simulink model "simsop"  (R2025a)
settings: Solver=VariableStepAuto  StartTime=0.0  StopTime=10.0  RelTol=1e-3
undefined symbols (not defined in the file or in its folder): dspblkCoreblockFVToolHelper, gcbh
libraries: simulink x3

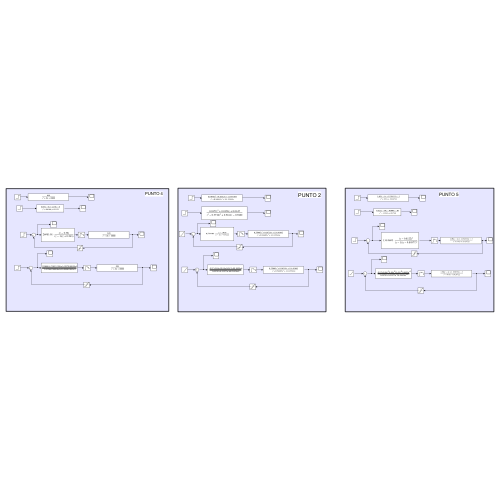
[thumbnail: Simulink's stored preview of the top-level diagram]
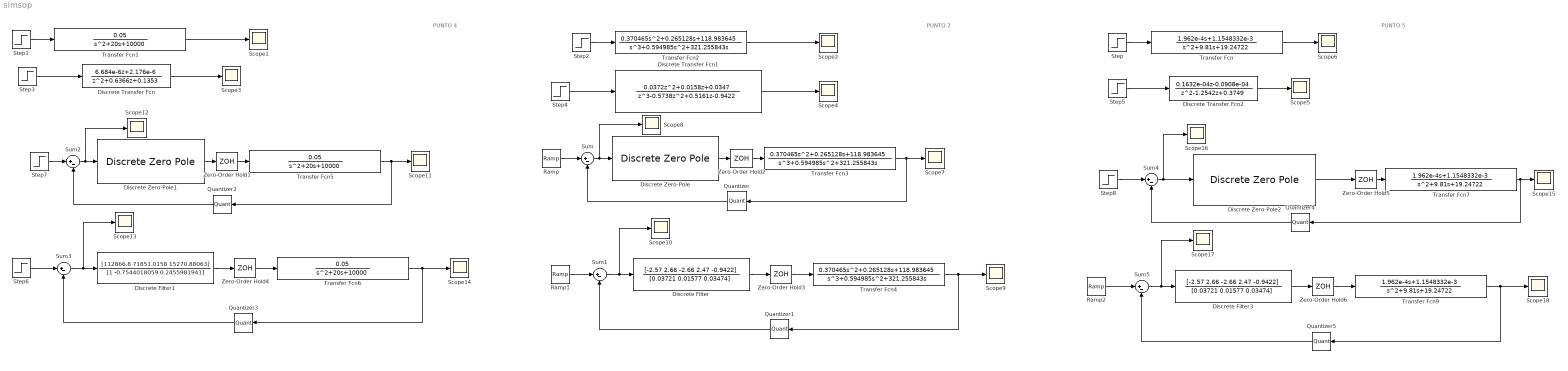
== system simsop ==
  note: PUNTO 5
  note: PUNTO 4
  note: PUNTO 2
  Discrete Transfer Fcn : DiscreteTransferFcn  LoadFcn=dspblkCoreblockFVToolHelper(gcbh,'load');  Numerator=[6.684e-6 2.176e-6]  Denominator=[1 0.6366 0.1353]
  Discrete Transfer Fcn1 : DiscreteTransferFcn  LoadFcn=dspblkCoreblockFVToolHelper(gcbh,'load');  Numerator="[0.0372    0.0158    0.0347]"  Denominator="[1   -0.5738    0.5161   -0.9422]"
  Discrete Transfer Fcn2 : DiscreteTransferFcn  LoadFcn=dspblkCoreblockFVToolHelper(gcbh,'load');  Numerator="[0.1632e-04   -0.0908e-04]"  Denominator="[1 -1.2542    0.3749]"
  Discrete Zero-Pole : DiscreteZeroPole  Zeros=[1.016]  Poles=[1 0.8222]  Gain=0.5798809  SampleTime=-1
  Discrete Zero-Pole1 : DiscreteZeroPole  Zeros=[2.52]  Poles=[1 -0.243]  Gain=26983.01  SampleTime=-1
  Discrete Zero-Pole2 : DiscreteZeroPole  Zeros=[0.8122 0.8122]  Poles=[1 0.80577 0.80577]  Gain=133.0695  SampleTime=-1
  Discrete Filter : DiscreteFilter  LoadFcn=dspblkCoreblockFVToolHelper(gcbh,'load');  Numerator=[-2.57 2.66 -2.66 2.47 -0.9422]  Denominator=[0.03721 0.01577 0.03474]
  Discrete Filter1 : DiscreteFilter  LoadFcn=dspblkCoreblockFVToolHelper(gcbh,'load');  Numerator=[112866.8 71851.0158 15270.88063]  Denominator=[1 -0.7544018059 0.2455981941]
  Discrete Filter3 : DiscreteFilter  LoadFcn=dspblkCoreblockFVToolHelper(gcbh,'load');  Numerator=[-2.57 2.66 -2.66 2.47 -0.9422]  Denominator=[0.03721 0.01577 0.03474]
  Quantizer{,1..5} (6 alike) : Quantizer  QuantizationInterval=3.3/1024
  Ramp : simulink/Sources/Ramp  slope=1  start=0  InitialOutput=0
  Ramp1 : simulink/Sources/Ramp  slope=1  start=0  InitialOutput=0
  Ramp2 : simulink/Sources/Ramp  slope=1  start=0  InitialOutput=0
  Scope{1..18} (18 alike) : Scope
  Step{,1..8} (9 alike) : Step  Time=0  SampleTime=0
  Sum{,1..5} (6 alike) : Sum  Inputs=|+-
  Transfer Fcn : TransferFcn  Numerator=[1.962e-4 1.1548332e-3]  Denominator=[1 9.81 19.24722]
  Transfer Fcn1 : TransferFcn  Numerator=[0.05]  Denominator=[1 20 10000]
  Transfer Fcn2 : TransferFcn  Numerator=[0.370465 0.265128 118.983645]  Denominator=[1 0.594985 321.255843 0]
  Transfer Fcn3 : TransferFcn  Numerator=[0.370465 0.265128 118.983645]  Denominator=[1 0.594985 321.255843 0]
  Transfer Fcn4 : TransferFcn  Numerator=[0.370465 0.265128 118.983645]  Denominator=[1 0.594985 321.255843 0]
  Transfer Fcn5 : TransferFcn  Numerator=[0.05]  Denominator=[1 20 10000]
  Transfer Fcn6 : TransferFcn  Numerator=[0.05]  Denominator=[1 20 10000]
  Transfer Fcn7 : TransferFcn  Numerator=[1.962e-4 1.1548332e-3]  Denominator=[1 9.81 19.24722]
  Transfer Fcn9 : TransferFcn  Numerator=[1.962e-4 1.1548332e-3]  Denominator=[1 9.81 19.24722]
  Zero-Order Hold{1..6} (6 alike) : ZeroOrderHold  SampleTime=0.1
  wires:
  Transfer Fcn/1 -> Scope6/1
  Step1/1 -> Transfer Fcn1/1
  Step2/1 -> Transfer Fcn2/1
  Discrete Transfer Fcn/1 -> Scope3/1
  Transfer Fcn1/1 -> Scope1/1
  Step3/1 -> Discrete Transfer Fcn/1
  Step4/1 -> Discrete Transfer Fcn1/1
  Transfer Fcn2/1 -> Scope2/1
  Discrete Transfer Fcn1/1 -> Scope4/1
  Discrete Transfer Fcn2/1 -> Scope5/1
  Discrete Zero-Pole/1 -> Zero-Order Hold2/1
  Quantizer/1 -> Sum/2
  Sum/1 -> Discrete Zero-Pole/1, Scope8/1
  Transfer Fcn3/1 -> Scope7/1, Quantizer/1
  Ramp/1 -> Sum/1
  Zero-Order Hold2/1 -> Transfer Fcn3/1
  Discrete Filter/1 -> Zero-Order Hold3/1
  Quantizer1/1 -> Sum1/2
  Zero-Order Hold3/1 -> Transfer Fcn4/1
  Sum1/1 -> Scope10/1, Discrete Filter/1
  Transfer Fcn4/1 -> Scope9/1, Quantizer1/1
  Ramp1/1 -> Sum1/1
  Zero-Order Hold1/1 -> Transfer Fcn5/1
  Step7/1 -> Sum2/1
  Transfer Fcn5/1 -> Quantizer2/1, Scope11/1
  Sum2/1 -> Scope12/1, Discrete Zero-Pole1/1
  Quantizer2/1 -> Sum2/2
  Discrete Zero-Pole1/1 -> Zero-Order Hold1/1
  Step6/1 -> Sum3/1
  Transfer Fcn6/1 -> Quantizer3/1, Scope14/1
  Sum3/1 -> Discrete Filter1/1, Scope13/1
  Zero-Order Hold4/1 -> Transfer Fcn6/1
  Quantizer3/1 -> Sum3/2
  Discrete Filter1/1 -> Zero-Order Hold4/1
  Discrete Filter3/1 -> Zero-Order Hold6/1
  Quantizer5/1 -> Sum5/2
  Zero-Order Hold6/1 -> Transfer Fcn9/1
  Sum5/1 -> Discrete Filter3/1, Scope17/1
  Transfer Fcn9/1 -> Scope18/1, Quantizer5/1
  Ramp2/1 -> Sum5/1
  Discrete Zero-Pole2/1 -> Zero-Order Hold5/1
  Quantizer4/1 -> Sum4/2
  Sum4/1 -> Scope16/1, Discrete Zero-Pole2/1
  Transfer Fcn7/1 -> Quantizer4/1, Scope15/1
  Step8/1 -> Sum4/1
  Zero-Order Hold5/1 -> Transfer Fcn7/1
  Step/1 -> Transfer Fcn/1
  Step5/1 -> Discrete Transfer Fcn2/1
